simulink model "Hopf_oscillator_2legs"  (R2021b)
settings: Solver=VariableStepAuto  StartTime=0.0  StopTime=10.0  RelTol=1e-3
undefined symbols (not defined in the file): A, alpha, delta_phi, epsilon, f, k, tau
settings Model: Creator=kaiget  LastModifiedBy=kaiget

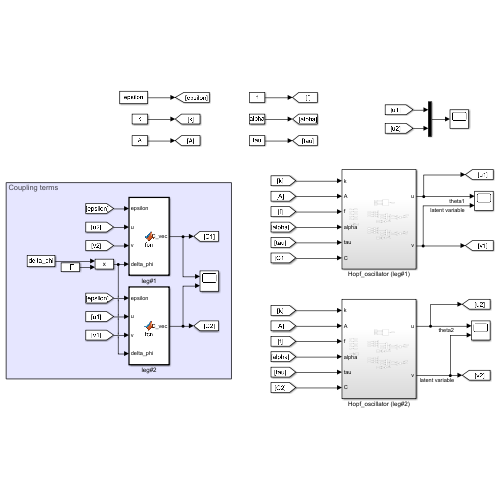
[thumbnail: Simulink's stored preview of the top-level diagram]
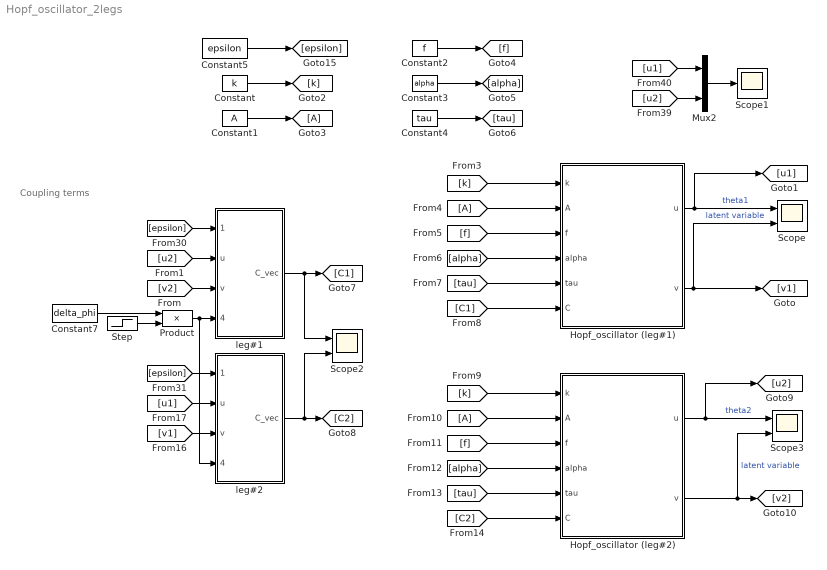
== system Hopf_oscillator_2legs ==
  note: Coupling terms
  Constant : Constant  Value=k
  Constant1 : Constant  Value=A
  Constant2 : Constant  Value=f
  Constant3 : Constant  Value=alpha
  Constant4 : Constant  Value=tau
  Constant5 : Constant  Value=epsilon
  Constant7 : Constant  Value=delta_phi
  Hopf_oscillator (leg#1) : Subsystem
  Hopf_oscillator (leg#2) : Subsystem
  Mux2 : Mux  Inputs=2
  Product : Product
  Scope : Scope  NumInputPorts=2
  Scope1 : Scope
  Scope2 : Scope  NumInputPorts=2
  Scope3 : Scope  NumInputPorts=2
  Step : Step  Time=5  Before=-1  After=2  SampleTime=0
  leg#1 : MATLAB Function  TreatAsAtomicUnit=on
  leg#2 : MATLAB Function  TreatAsAtomicUnit=on
  wires:
  [epsilon] -> leg#2/1(epsilon)
  [epsilon] -> leg#1/1(epsilon)
  [u2] -> leg#1/2(u)
  [v2] -> leg#1/3(v)
  [v1] -> leg#2/3(v)
  leg#1/1(C_vec) -> [C1], Scope2/1
  leg#2/1(C_vec) -> [C2], Scope2/2
  Product/1 -> leg#2/4(delta_phi), leg#1/4(delta_phi)
  [u1] -> leg#2/2(u)
  Step/1 -> Product/2
  Constant7/1 -> Product/1
  Hopf_oscillator (leg#1)/1(u) -> [u1], Scope/1  "theta1"
  [alpha] -> Hopf_oscillator (leg#2)/4(alpha)
  [f] -> Hopf_oscillator (leg#2)/3(f)
  Hopf_oscillator (leg#2)/1(u) -> [u2], Scope3/1  "theta2"
  [C2] -> Hopf_oscillator (leg#2)/6(C)
  [k] -> Hopf_oscillator (leg#2)/1(k)
  [tau] -> Hopf_oscillator (leg#1)/5(tau)
  [A] -> Hopf_oscillator (leg#2)/2(A)
  [f] -> Hopf_oscillator (leg#1)/3(f)
  [alpha] -> Hopf_oscillator (leg#1)/4(alpha)
  Hopf_oscillator (leg#2)/2(v) -> [v2], Scope3/2  "latent variable"
  [tau] -> Hopf_oscillator (leg#2)/5(tau)
  Hopf_oscillator (leg#1)/2(v) -> [v1], Scope/2  "latent variable"
  [A] -> Hopf_oscillator (leg#1)/2(A)
  [C1] -> Hopf_oscillator (leg#1)/6(C)
  [k] -> Hopf_oscillator (leg#1)/1(k)
  Constant5/1 -> [epsilon]
  Constant4/1 -> [tau]
  Constant1/1 -> [A]
  Constant3/1 -> [alpha]
  Constant/1 -> [k]
  Constant2/1 -> [f]
  [u1] -> Mux2/1
  Mux2/1 -> Scope1/1
  [u2] -> Mux2/2

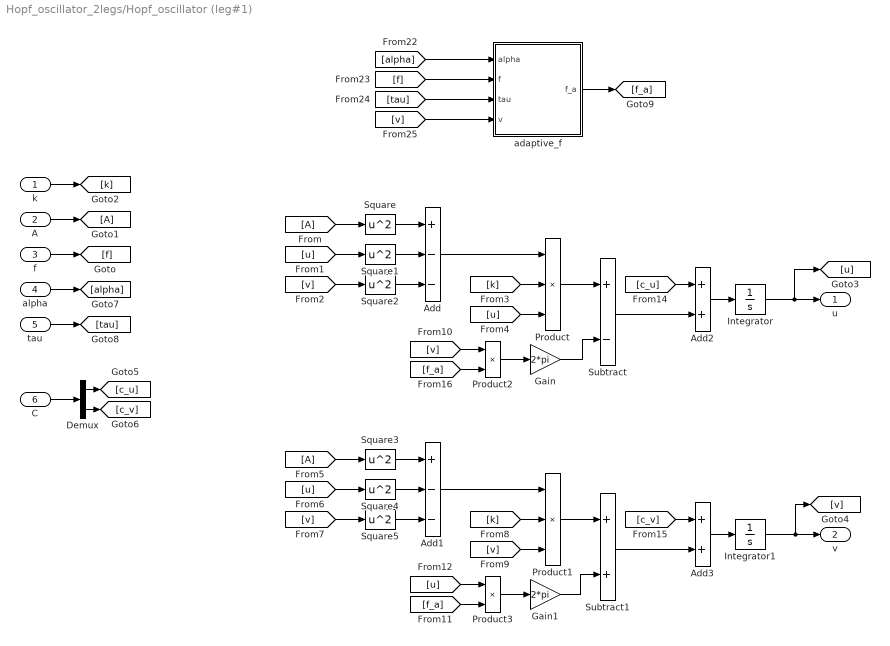
== system Hopf_oscillator_2legs/Hopf_oscillator (leg#1) ==
  k : Inport
  A : Inport  Port=2
  f : Inport  Port=3
  alpha : Inport  Port=4
  tau : Inport  Port=5
  C : Inport  Port=6
  Add : Sum  Inputs=+--
  Add1 : Sum  Inputs=+--
  Add2 : Sum
  Add3 : Sum
  Demux : Demux  Outputs=2
  Gain : Gain  Gain=2*pi
  Gain1 : Gain  Gain=2*pi
  Integrator : Integrator  InitialCondition=0.5
  Integrator1 : Integrator  InitialCondition=0.5
  Product : Product  Inputs=3
  Product1 : Product  Inputs=3
  Product2 : Product
  Product3 : Product
  Square{,1..5} (6 alike) : Math  Operator=square  SaturateOnIntegerOverflow=on
  Subtract : Sum  Inputs=+-
  Subtract1 : Sum
  adaptive_f : MATLAB Function  TreatAsAtomicUnit=on
  u : Outport
  v : Outport  Port=2
  wires:
  Integrator/1 -> [u], u/1
  f/1 -> [f]
  A/1 -> [A]
  k/1 -> [k]
  Integrator1/1 -> [v], v/1
  [A] -> Square/1
  [u] -> Square1/1
  [v] -> Square2/1
  Square2/1 -> Add/3
  Square1/1 -> Add/2
  Square/1 -> Add/1
  Add/1 -> Product/1
  [k] -> Product/2
  [u] -> Product/3
  Product/1 -> Subtract/1
  Square3/1 -> Add1/1
  Square4/1 -> Add1/2
  Square5/1 -> Add1/3
  [v] -> Product1/3
  Product1/1 -> Subtract1/1
  [v] -> Square5/1
  [A] -> Square3/1
  [u] -> Square4/1
  Add1/1 -> Product1/1
  [k] -> Product1/2
  [v] -> Product2/1
  [f_a] -> Product2/2
  Product2/1 -> Gain/1
  Gain/1 -> Subtract/2
  [u] -> Product3/1
  Product3/1 -> Gain1/1
  [f_a] -> Product3/2
  Gain1/1 -> Subtract1/2
  Subtract/1 -> Add2/2
  C/1 -> Demux/1
  Demux/1 -> [c_u]
  Demux/2 -> [c_v]
  [c_u] -> Add2/1
  Add2/1 -> Integrator/1
  Subtract1/1 -> Add3/2
  [c_v] -> Add3/1
  Add3/1 -> Integrator1/1
  alpha/1 -> [alpha]
  tau/1 -> [tau]
  [alpha] -> adaptive_f/1(alpha)
  [f] -> adaptive_f/2(f)
  [tau] -> adaptive_f/3(tau)
  [v] -> adaptive_f/4(v)
  adaptive_f/1(f_a) -> [f_a]

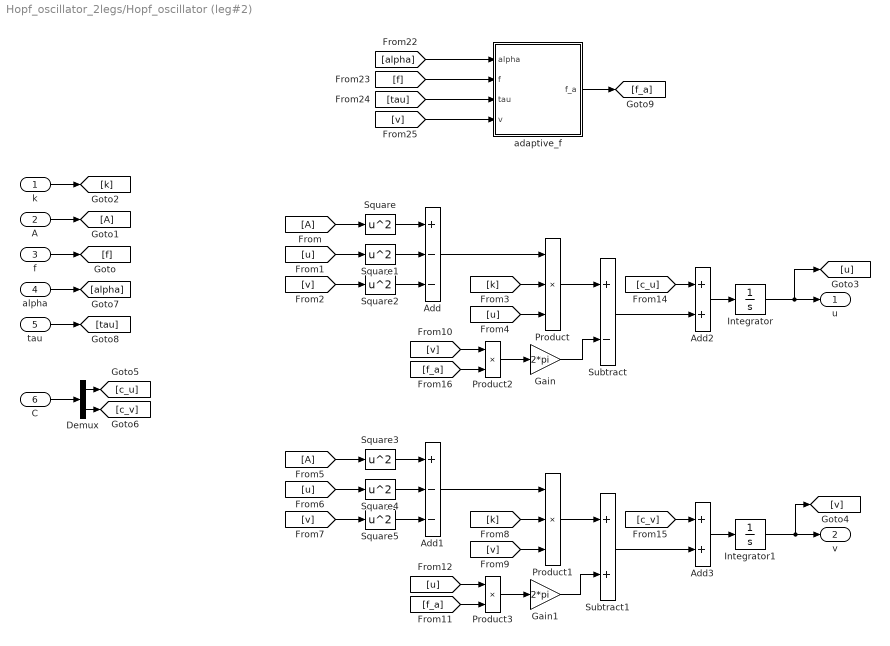
== system Hopf_oscillator_2legs/Hopf_oscillator (leg#2) ==
  k : Inport
  A : Inport  Port=2
  f : Inport  Port=3
  alpha : Inport  Port=4
  tau : Inport  Port=5
  C : Inport  Port=6
  Add : Sum  Inputs=+--
  Add1 : Sum  Inputs=+--
  Add2 : Sum
  Add3 : Sum
  Demux : Demux  Outputs=2
  Gain : Gain  Gain=2*pi
  Gain1 : Gain  Gain=2*pi
  Integrator : Integrator  InitialCondition=1
  Integrator1 : Integrator  InitialCondition=1
  Product : Product  Inputs=3
  Product1 : Product  Inputs=3
  Product2 : Product
  Product3 : Product
  Square{,1..5} (6 alike) : Math  Operator=square  SaturateOnIntegerOverflow=on
  Subtract : Sum  Inputs=+-
  Subtract1 : Sum
  adaptive_f : MATLAB Function  TreatAsAtomicUnit=on
  u : Outport
  v : Outport  Port=2
  wires:
  Integrator/1 -> [u], u/1
  f/1 -> [f]
  A/1 -> [A]
  k/1 -> [k]
  Integrator1/1 -> [v], v/1
  [A] -> Square/1
  [u] -> Square1/1
  [v] -> Square2/1
  Square2/1 -> Add/3
  Square1/1 -> Add/2
  Square/1 -> Add/1
  Add/1 -> Product/1
  [k] -> Product/2
  [u] -> Product/3
  Product/1 -> Subtract/1
  Square3/1 -> Add1/1
  Square4/1 -> Add1/2
  Square5/1 -> Add1/3
  [v] -> Product1/3
  Product1/1 -> Subtract1/1
  [v] -> Square5/1
  [A] -> Square3/1
  [u] -> Square4/1
  Add1/1 -> Product1/1
  [k] -> Product1/2
  [v] -> Product2/1
  [f_a] -> Product2/2
  Product2/1 -> Gain/1
  Gain/1 -> Subtract/2
  [u] -> Product3/1
  Product3/1 -> Gain1/1
  [f_a] -> Product3/2
  Gain1/1 -> Subtract1/2
  Subtract/1 -> Add2/2
  C/1 -> Demux/1
  Demux/1 -> [c_u]
  Demux/2 -> [c_v]
  [c_u] -> Add2/1
  Add2/1 -> Integrator/1
  Subtract1/1 -> Add3/2
  [c_v] -> Add3/1
  Add3/1 -> Integrator1/1
  alpha/1 -> [alpha]
  tau/1 -> [tau]
  [alpha] -> adaptive_f/1(alpha)
  [f] -> adaptive_f/2(f)
  [tau] -> adaptive_f/3(tau)
  [v] -> adaptive_f/4(v)
  adaptive_f/1(f_a) -> [f_a]

== matlab function Hopf_oscillator_2legs/Hopf_oscillator (leg#2)/adaptive_f ==
  data: alpha input; f_a output; f input; tau input; v input
 % calculate the adaptive frequency f through (4) in 
 % 'Design and Locomotion Control of a Biomimetic Underwater Vehicle ... '
function f_a = adaptive_f(alpha, f, tau, v)
    f1 = f/2/alpha;
    f2 = (2*alpha - 1)*f/(2*alpha*(1 - alpha)*(1 + exp(-tau*v)));
    f_a = f1 + f2;

== matlab function Hopf_oscillator_2legs/Hopf_oscillator (leg#1)/adaptive_f ==
  data: alpha input; f_a output; f input; tau input; v input
 % calculate the adaptive frequency f through (4) in 
 % 'Design and Locomotion Control of a Biomimetic Underwater Vehicle ... '
function f_a = adaptive_f(alpha, f, tau, v)
    f1 = f/2/alpha;
    f2 = (2*alpha - 1)*f/(2*alpha*(1 - alpha)*(1 + exp(-tau*v)));
    f_a = f1 + f2;

== matlab function Hopf_oscillator_2legs/leg#1 ==
  data: epsilon input; u input; C_vec output; v input; delta_phi input
function C_vec = fcn(epsilon, u, v, delta_phi)
    C1 = 0;
    C2 = epsilon*(-u*sin(delta_phi) + v*cos(delta_phi));
    C_vec = [C1; C2];

== matlab function Hopf_oscillator_2legs/leg#2 ==
  data: epsilon input; u input; C_vec output; v input; delta_phi input
function C_vec = fcn(epsilon, u, v, delta_phi)
    C1 = 0;
    C2 = epsilon*(u*sin(delta_phi) + v*cos(delta_phi));
    C_vec = [C1; C2];
